simulink model "Controller"  (R2018b)
settings: Solver=FixedStepAuto  StartTime=0.0  StopTime=15  RelTol=1e-3  EnableMultiTasking=on
undefined symbols (not defined in the file): A, B, C, K, K_z, Ke, L, Ld, sysSS, sysSSD
libraries: legoev3lib x2
settings Model: ExtModeTrigDuration=2  Creator=stinu  LastModifiedBy=stinu
settings SolverCC: PositivePriorityOrder=on
settings OptimizationCC: EnhancedBackFolding=on  PassReuseOutputArgsAs=Individual arguments  MaxStackSize=64  OptimizeBlockOrder=speed  DifferentSizesBufferReuse=on  OptimizationCustomize=off
settings DebuggingCC: ParameterTunabilityLossMsg=error
settings HardwareCC: ProdBitPerPointer=32  ProdBitPerSizeT=32  ProdBitPerPtrDiffT=32  ProdLargestAtomicInteger=Long  ProdWordSize=32  ProdHWDeviceType=ARM Compatible->ARM 9  UseEmbeddedCoderFeatures=off  UseSimulinkCoderFeatures=off
settings SFSimCC: MATLABDynamicMemAlloc=off
settings RTWCC: SystemTargetFile=ert.tlc  HardwareBoard=LEGO MINDSTORMS EV3  TLCOptions="-aInlineSetEventsForThisBaseRateFcn=TLC_FALSE -aSuppressMultiTaskScheduler=TLC_FALSE  -aRateBasedStepFcn=0"  TemplateMakefile=ert_default_tmf  GenerateReport=on  Toolchain=Sourcery G++ Lite v2009q3  IncludeHyperlinkInReport=on  LaunchReport=on  GenerateTraceInfo=on  GenerateTraceReport=on  GenerateTraceReportSl=on  GenerateTraceReportSf=on  GenerateTraceReportEml=on
settings CodeAppCC: ForceParamTrailComments=on  IgnoreCustomStorageClasses=off  OperatorAnnotations=on  SimulinkDataObjDesc=on  SFDataObjDesc=on  InsertBlockDesc=on
settings ERTTargetCC: SupportContinuousTime=on  SupportNonInlinedSFcns=on  SupportVariableSizeSignals=on

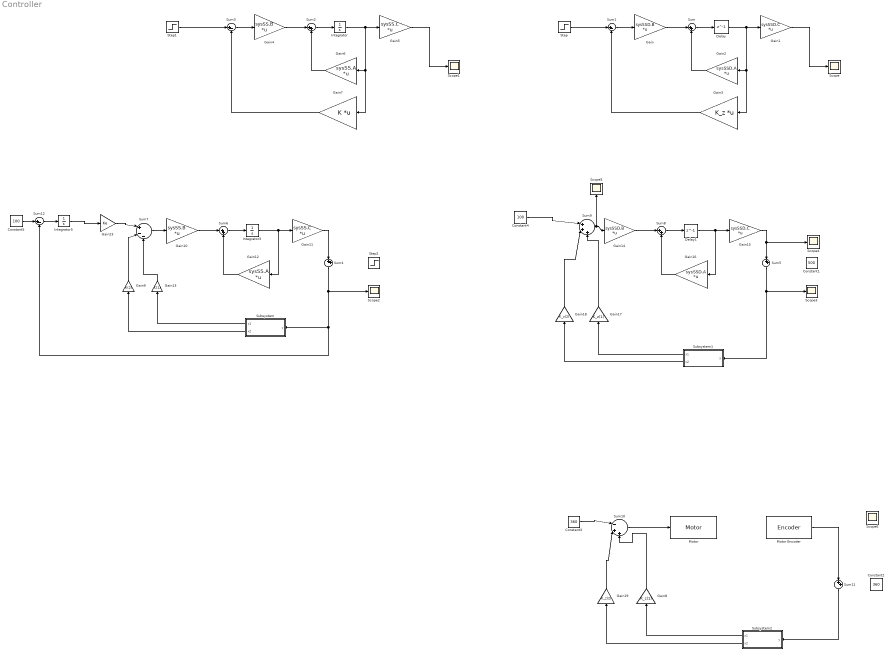
== system Controller ==
  Constant1 : Constant  Value=500
  Constant2 : Constant  Value=360
  Constant3 : Constant  Value=360
  Constant4 : Constant  Value=100
  Constant5 : Constant  Value=100
  Delay : Delay  DelayLength=1  InitialCondition=0
  Delay1 : Delay  DelayLength=1  InitialCondition=0
  Gain : Gain  Gain=sysSSD.B  Multiplication=Matrix(K*u)
  Gain1 : Gain  Gain=sysSSD.C  Multiplication=Matrix(K*u)
  Gain10 : Gain  Gain=sysSS.B  Multiplication=Matrix(K*u)
  Gain11 : Gain  Gain=sysSS.C  Multiplication=Matrix(K*u)
  Gain12 : Gain  Gain=sysSS.A  Multiplication=Matrix(K*u)
  Gain13 : Gain  Gain=K(1)
  Gain14 : Gain  Gain=sysSSD.B  Multiplication=Matrix(K*u)
  Gain15 : Gain  Gain=sysSSD.C  Multiplication=Matrix(K*u)
  Gain16 : Gain  Gain=sysSSD.A  Multiplication=Matrix(K*u)
  Gain17 : Gain  Gain=K_z(1)
  Gain18 : Gain  Gain=K_z(2)
  Gain19 : Gain  Gain=K_z(2)
  Gain2 : Gain  Gain=sysSSD.A  Multiplication=Matrix(K*u)
  Gain23 : Gain  Gain=Ke
  Gain3 : Gain  Gain=K_z  Multiplication=Matrix(K*u)
  Gain4 : Gain  Gain=sysSS.B  Multiplication=Matrix(K*u)
  Gain5 : Gain  Gain=sysSS.C  Multiplication=Matrix(K*u)
  Gain6 : Gain  Gain=sysSS.A  Multiplication=Matrix(K*u)
  Gain7 : Gain  Gain=K  Multiplication=Matrix(K*u)
  Gain8 : Gain  Gain=K_z(1)
  Gain9 : Gain  Gain=K(2)
  Integrator : Integrator
  Integrator3 : Integrator
  Integrator5 : Integrator
  Motor : legoev3lib/Motor  sportNumber=A  sstopAction=Brake
  Motor Encoder : legoev3lib/Encoder  portNumber=A  opMode=No reset  sampleTime=0.01
      settings: SourceProductName=Simulink Support Package for LEGO MINDSTORMS EV3 Hardware  SourceProductBaseCode=LEGOEV3
  Scope{,1..6} (7 alike) : Scope
  Step : Step  After=100  SampleTime=0.01
  Step1 : Step
  Step2 : Step  Time=5  After=100
  Subsystem : Subsystem
  Subsystem1 : Subsystem
  Subsystem2 : Subsystem
  Sum{,2,4..6,8,11} (7 alike) : Sum  Inputs=|++
  Sum1 : Sum  Inputs=|+-
  Sum10 : Sum  Inputs=|-++
  Sum12 : Sum  Inputs=|+-
  Sum3 : Sum  Inputs=|+-
  Sum7 : Sum  Inputs=|+--
  Sum9 : Sum  Inputs=|+++
  wires:
  Delay/1 -> Gain3/1, Gain2/1, Gain1/1
  Sum/1 -> Delay/1
  Gain/1 -> Sum/1
  Gain2/1 -> Sum/2
  Gain3/1 -> Sum1/2
  Sum1/1 -> Gain/1
  Step/1 -> Sum1/1
  Gain1/1 -> Scope/1
  Gain5/1 -> Scope1/1
  Gain7/1 -> Sum3/2
  Sum3/1 -> Gain4/1
  Sum2/1 -> Integrator/1
  Integrator/1 -> Gain7/1, Gain6/1, Gain5/1
  Gain4/1 -> Sum2/1
  Gain6/1 -> Sum2/2
  Integrator3/1 -> Gain12/1, Gain11/1
  Gain12/1 -> Sum6/2
  Sum6/1 -> Integrator3/1
  Sum7/1 -> Gain10/1
  Gain10/1 -> Sum6/1
  Subsystem/1(x1) -> Gain13/1
  Subsystem/2(x2) -> Gain9/1
  Gain13/1 -> Sum7/3
  Gain9/1 -> Sum7/2
  Gain11/1 -> Sum4/1
  Sum4/1 -> Scope2/1, Sum12/2, Subsystem/1(y)
  Subsystem1/2(x2) -> Gain18/1
  Gain14/1 -> Sum8/1
  Gain16/1 -> Sum8/2
  Gain15/1 -> Sum5/1, Scope4/1
  Gain17/1 -> Sum9/3
  Sum5/1 -> Scope3/1, Subsystem1/1(y)
  Gain18/1 -> Sum9/2
  Subsystem1/1(x1) -> Gain17/1
  Delay1/1 -> Gain16/1, Gain15/1
  Sum9/1 -> Scope5/1, Gain14/1
  Sum8/1 -> Delay1/1
  Subsystem2/1(x1) -> Gain8/1
  Subsystem2/2(x2) -> Gain19/1
  Gain19/1 -> Sum10/2
  Gain8/1 -> Sum10/3
  Sum10/1 -> Motor/1
  Motor Encoder/1 -> Sum11/1
  Sum11/1 -> Subsystem2/1(y)
  Step1/1 -> Sum3/1
  Constant3/1 -> Sum10/1
  Integrator5/1 -> Gain23/1
  Gain23/1 -> Sum7/1
  Constant5/1 -> Sum12/1
  Sum12/1 -> Integrator5/1
  Constant4/1 -> Sum9/1

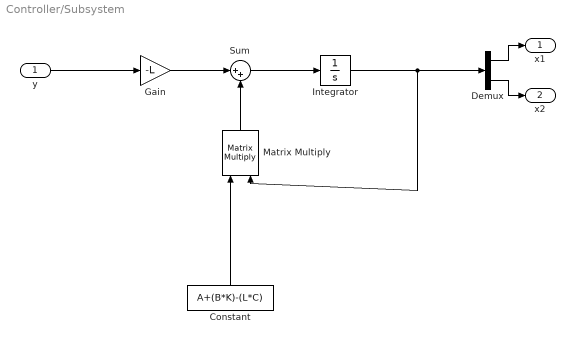
== system Controller/Subsystem ==
  y : Inport
  Constant : Constant  Value=A+(B*K)-(L*C)
  Demux : Demux  Outputs=2
  Gain : Gain  Gain=-L
  Integrator : Integrator
  Matrix Multiply : Product  Multiplication=Matrix(*)
  Sum : Sum  Inputs=|++
  x1 : Outport
  x2 : Outport  Port=2
  wires:
  y/1 -> Gain/1
  Gain/1 -> Sum/1
  Sum/1 -> Integrator/1
  Integrator/1 -> Matrix Multiply/2, Demux/1
  Matrix Multiply/1 -> Sum/2
  Demux/1 -> x1/1
  Demux/2 -> x2/1
  Constant/1 -> Matrix Multiply/1

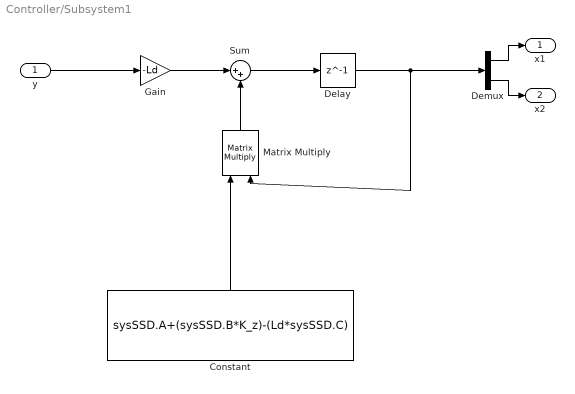
== system Controller/Subsystem1 ==
  y : Inport
  Constant : Constant  Value=sysSSD.A+(sysSSD.B*K_z)-(Ld*sysSSD.C)
  Delay : Delay  DelayLength=1  InitialCondition=0
  Demux : Demux  Outputs=2
  Gain : Gain  Gain=-Ld
  Matrix Multiply : Product  Multiplication=Matrix(*)
  Sum : Sum  Inputs=|++
  x1 : Outport
  x2 : Outport  Port=2
  wires:
  y/1 -> Gain/1
  Gain/1 -> Sum/1
  Sum/1 -> Delay/1
  Matrix Multiply/1 -> Sum/2
  Demux/1 -> x1/1
  Demux/2 -> x2/1
  Constant/1 -> Matrix Multiply/1
  Delay/1 -> Matrix Multiply/2, Demux/1

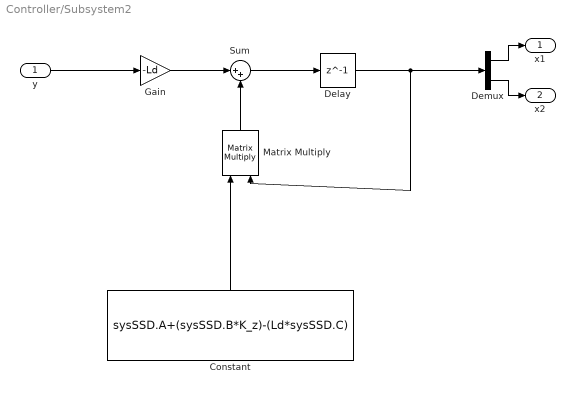
== system Controller/Subsystem2 ==
  y : Inport
  Constant : Constant  Value=sysSSD.A+(sysSSD.B*K_z)-(Ld*sysSSD.C)
  Delay : Delay  DelayLength=1  InitialCondition=0
  Demux : Demux  Outputs=2
  Gain : Gain  Gain=-Ld
  Matrix Multiply : Product  Multiplication=Matrix(*)
  Sum : Sum  Inputs=|++
  x1 : Outport
  x2 : Outport  Port=2
  wires:
  y/1 -> Gain/1
  Gain/1 -> Sum/1
  Sum/1 -> Delay/1
  Matrix Multiply/1 -> Sum/2
  Demux/1 -> x1/1
  Demux/2 -> x2/1
  Constant/1 -> Matrix Multiply/1
  Delay/1 -> Matrix Multiply/2, Demux/1
